simulink subsystem "Szakasz"  (R2024b)
settings: Solver=VariableStepAuto  StartTime=0.0  StopTime=10.0  RelTol=1e-3
libraries: mobileRoboticsLib x1
settings Model: Creator=Asus  LastModifiedBy=Asus

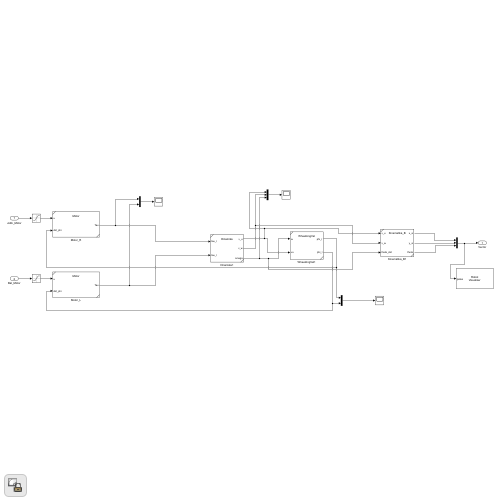
[thumbnail: Simulink's stored preview of the top-level diagram]
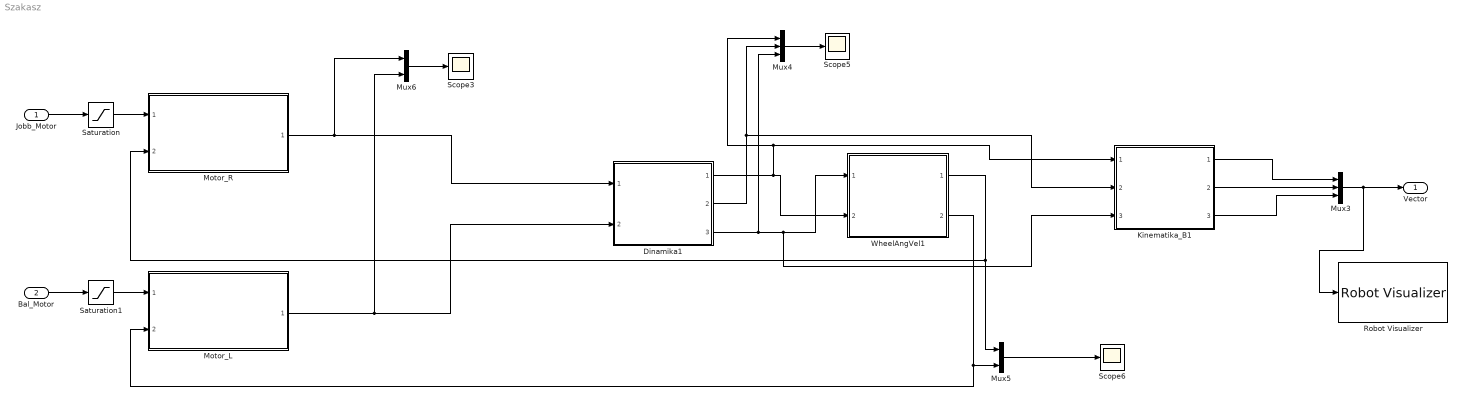
== system Szakasz ==
  Jobb_Motor : Inport
  Bal_Motor : Inport  Port=2
  Dinamika1 : Subsystem  ReferencedSubsystem=Dinamika
  Kinematika_B1 : Subsystem  ReferencedSubsystem=Kinematika_B
  Motor_L : Subsystem  ReferencedSubsystem=Motor
  Motor_R : Subsystem  ReferencedSubsystem=Motor
  Mux3 : Mux  Inputs=3
  Mux4 : Mux  Inputs=3
  Mux5 : Mux  Inputs=2
  Mux6 : Mux  Inputs=2
  Robot Visualizer : mobileRoboticsLib/Environments/Robot Visualizer  robotRadius=L  showTrajectory=on  hasWaypoints=off  hasLidar=off  sensorOffset=[ 0, 0 ]  scanAngles=[ -pi/4, 0, pi/4 ]  hasObjDetector=off  objDetectorOffset=[ 0, 0 ]  objDetectorAngle=0  objDetectorFOV=pi/4  objDetectorMaxRange=5  objectColors=[ 1, 0, 0; 0, 1, 0; 0, 0, 1 ]  objectMarkers=s
  Saturation : Saturate  UpperLimit=5  LowerLimit=-5
  Saturation1 : Saturate  UpperLimit=5  LowerLimit=-5
  Scope3 : Scope
  Scope5 : Scope
  Scope6 : Scope
  WheelAngVel1 : Subsystem  ReferencedSubsystem=WheelAngVel
  Vector : Outport
  wires:
  Jobb_Motor/1 -> Saturation/1
  Kinematika_B1/1 -> Mux3/1
  Dinamika1/2 -> Mux4/2, Kinematika_B1/2
  Mux6/1 -> Scope3/1
  WheelAngVel1/2 -> Mux5/2, Motor_L/2
  Kinematika_B1/3 -> Mux3/3
  Dinamika1/3 -> WheelAngVel1/1, Kinematika_B1/3, Mux4/3
  Mux5/1 -> Scope6/1
  Motor_R/1 -> Dinamika1/1, Mux6/1
  Mux4/1 -> Scope5/1
  Saturation/1 -> Motor_R/1
  WheelAngVel1/1 -> Motor_R/2, Mux5/1
  Motor_L/1 -> Dinamika1/2, Mux6/2
  Saturation1/1 -> Motor_L/1
  Dinamika1/1 -> WheelAngVel1/2, Kinematika_B1/1, Mux4/1
  Kinematika_B1/2 -> Mux3/2
  Bal_Motor/1 -> Saturation1/1
  Mux3/1 -> Vector/1, Robot Visualizer/1
